simulink model "PLANTA_2019"  (R2020a)
settings: Solver=FixedStepAuto  StartTime=0.0  StopTime=10  FixedStep=0.1  RelTol=1e-3
libraries: simulink x1
settings Model: SimulationMode=accelerator  Creator=Alex  LastModifiedBy=marco
settings SFSimCC: CustomCodeUndefinedFunction=UseInterfaceOnly

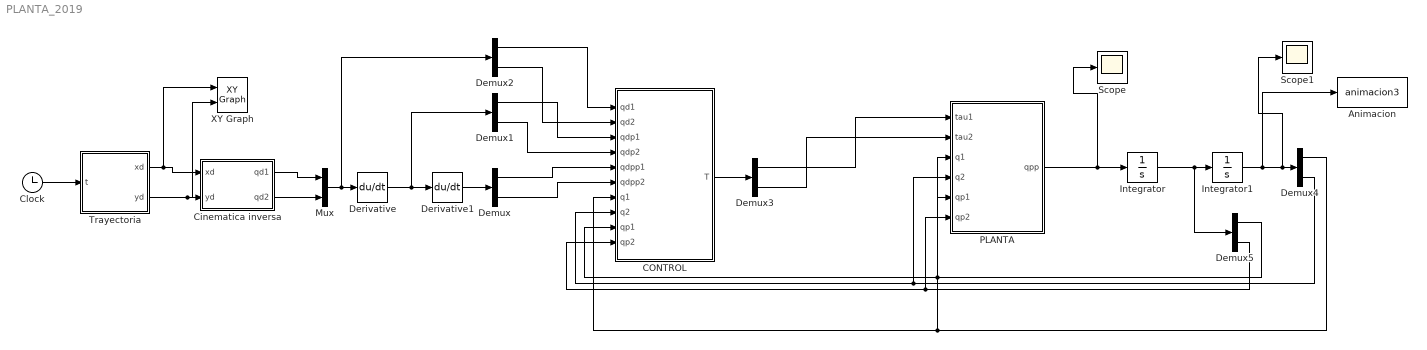
== system PLANTA_2019 ==
  Animacion : MATLABFcn  MATLABFcn=animacion3  OutputDimensions=0
  CONTROL : MATLAB Function  TreatAsAtomicUnit=on
  Cinematica inversa : MATLAB Function  TreatAsAtomicUnit=on
  Clock : Clock
  Demux{,1..5} (6 alike) : Demux  Outputs=2
  Derivative : Derivative
  Derivative1 : Derivative
  Integrator : Integrator  InitialCondition=[0 0]
  Integrator1 : Integrator  InitialCondition=[0 0]
  Mux : Mux  Inputs=2
  PLANTA : MATLAB Function  TreatAsAtomicUnit=on
  Scope : Scope
  Scope1 : Scope
  Trayectoria : MATLAB Function  TreatAsAtomicUnit=on
  XY Graph : simulink/Sinks/XY Graph  xmin=-1  xmax=1  ymin=-1  ymax=1  st=-1
  wires:
  PLANTA/1(qpp) -> Scope/1, Integrator/1
  Integrator/1 -> Demux5/1, Integrator1/1
  Clock/1 -> Trayectoria/1(t)
  Trayectoria/2(yd) -> XY Graph/2, Cinematica inversa/2(yd)
  Trayectoria/1(xd) -> Cinematica inversa/1(xd), XY Graph/1
  Cinematica inversa/1(qd1) -> Mux/1
  Mux/1 -> Demux2/1, Derivative/1
  Derivative/1 -> Demux1/1, Derivative1/1
  Derivative1/1 -> Demux/1
  Demux/1 -> CONTROL/5(qdpp1)
  Demux/2 -> CONTROL/6(qdpp2)
  Demux1/1 -> CONTROL/3(qdp1)
  Demux1/2 -> CONTROL/4(qdp2)
  Demux2/1 -> CONTROL/1(qd1)
  Demux2/2 -> CONTROL/2(qd2)
  CONTROL/1(T) -> Demux3/1
  Demux3/1 -> PLANTA/1(tau1)
  Demux3/2 -> PLANTA/2(tau2)
  Demux4/1 -> PLANTA/3(q1), CONTROL/7(q1)
  Demux4/2 -> PLANTA/4(q2), CONTROL/8(q2)
  Demux5/1 -> PLANTA/5(qp1), CONTROL/9(qp1)
  Demux5/2 -> PLANTA/6(qp2), CONTROL/10(qp2)
  Integrator1/1 -> Animacion/1, Scope1/1, Demux4/1
  Cinematica inversa/2(qd2) -> Mux/2

== matlab function PLANTA_2019/Trayectoria ==
  data: t input; xd output; yd output
function [xd,yd] = fcn(t)
% a=0.15;
% R=0.2;
% n=3;
% hx=0.3;
% hy=0.1;
% T=10;
% f=1/T;
% w=2*pi*f;
% xd=hx+(a+R*cos(n*w*t)^2)*cos(w*t);
% yd=hy+(a+R*cos(n*w*t)^2)*sin(w*t);

a=0.15;
R=0.2;
hx=0.2;
hy=0;
T=10;
f=1/T;
w=2*pi*f;
xd=hx+a*cos(w*t)/(1+sin(w*t)^2);
yd=hy+a*sin(w*t)*cos(w*t)/(1+sin(w*t)^2);

== matlab function PLANTA_2019/PLANTA ==
  data: tau1 input; qpp output; tau2 input; q1 input; q2 input; qp1 input; qp2 input
function qpp = fcn(tau1,tau2,q1,q2,qp1,qp2)
%Parámetros del primer eslabon

m1 = 0.067  %Masa de la barra 1(kg)
m2 =0.067  %Masa de la barra 2 (kg)
l1 = 0.3  % Longitud de la barra 1 (m)
lc1 = 0.14  % Longitud al centro de masa de la barra 2 (m)

l2= 0.3 %0Longitud de la baraa 2 (m)
lc2=0.15 %Longitud al centro de masa de la barra 2(m)
b1 = 0.0017  % Coeficiente de fricción viscosa de la barra 1
b2= 0.0013 %Coeficiente de fricción viscosa de la barra 2
g = 9.81  % Aceleración de la gravedad en la Tierra
I1 = 0.15  % Tensor de inercia del péndulo 1
I2= 0.14 %Tensor de inercia del péndulo 2

%Matriz de masas
M11=m1*lc1^2+m2*l2^2+m2*lc2^2+2*m2*l1*lc2*cos(q2)+I1+I2;
M12=m2*lc2^2+m2*l1*lc2*cos(q2)+I2;
M21=m2*lc2^2+m2*l1*lc2*cos(q2)+I2;
M22=m2*lc2^2+I2;
M=[M11 M12;M21 M22];

%Matriz de Coriollis
C11=-2*m2*l1*lc2*sin(q2)*qp2;
C12=-m2*l1*lc2*sin(q2)*qp2;
C21=m2*l1*lc2*sin(q2)*qp1;
C22=0
C=[C11 C12;C21 C22];

B11=b1;
B12=0;
B21=0;
B22=b2;
B=[B11 B12;B21 B22];

%Vector de gravedad
G1=(m1*lc1+m2*l1)*g*sin(q1)+m2*g*lc2*sin(q1+q2);
G2=m2*g*lc2*sin(q1+q2);

G=[G1;G2];

%Vector de posicion
q=[q1;q2];

%Vector de velocidad
qp=[qp1;qp2];

%Vector de entradas
%tau1=10;tau2=2;
T=[tau1;tau2]


%Planta

qpp = M\(T-C*qp-B*qp-G);

== matlab function PLANTA_2019/Cinematica inversa ==
  data: xd input; qd1 output; yd input; qd2 output
function [qd1,qd2] = fcn(xd,yd)
l1=0.3;
l2=0.3;
cosq2=(xd^2+yd^2-l1^2-l2^2)/(2*l1*l2);
qd2=atan2(sqrt(1-cosq2^2),cosq2);

qd1 = atan2(xd,-yd)-atan2(l2*sin(qd2),(l1+l2*cos(qd2)));

== matlab function PLANTA_2019/CONTROL ==
  data: qd1 input; T output; qd2 input; qdp1 input; qdp2 input; qdpp1 input; qdpp2 input; q1 input; q2 input; qp1 input; qp2 input
function T = fcn(qd1,qd2,qdp1,qdp2,qdpp1,qdpp2,q1,q2,qp1,qp2)
%Control por par calculado

m1 = 0.067  %Masa de la barra 1(kg)
m2 =0.067  %Masa de la barra 2 (kg)
l1 = 0.3  % Longitud de la barra 1 (m)
lc1 = 0.14  % Longitud al centro de masa de la barra 2 (m)

l2= 0.3 %0Longitud de la baraa 2 (m)
lc2=0.15 %Longitud al centro de masa de la barra 2(m)
b1 = 0.0017  % Coeficiente de fricción viscosa de la barra 1
b2= 0.0013 %Coeficiente de fricción viscosa de la barra 2
g = 9.81  % Aceleración de la gravedad en la Tierra
I1 = 0.15  % Tensor de inercia del péndulo 1
I2= 0.14 %Tensor de inercia del péndulo 2

%Matriz de masas
M11=m1*lc1^2+m2*l2^2+m2*lc2^2+2*m2*l1*lc2*cos(q2)+I1+I2;
M12=m2*lc2^2+m2*l1*lc2*cos(q2)+I2;
M21=m2*lc2^2+m2*l1*lc2*cos(q2)+I2;
M22=m2*lc2^2+I2;
M=[M11 M12;M21 M22];

%Matriz de Coriollis
C11=-2*m2*l1*lc2*sin(q2)*qp2;
C12=-m2*l1*lc2*sin(q2)*qp2;
C21=m2*l1*lc2*sin(q2)*qp1;
C22=0
C=[C11 C12;C21 C22];

B11=b1;
B12=0;
B21=0;
B22=b2;
B=[B11 B12;B21 B22];

%Vector de gravedad
G1=(m1*lc1+m2*l1)*g*sin(q1)+m2*g*lc2*sin(q1+q2);
G2=m2*g*lc2*sin(q1+q2);

G=[G1;G2];

%Vector de posicion
q=[q1;q2];

%Vector de velocidad
qp=[qp1;qp2];


kp1=15;
kp2=5;
kd1=3;
kd2=4;

%Ganancias

Kp11=kp1;
Kp12=0;
Kp21=0;
Kp22=kp2;
Kp=[Kp11 Kp12;Kp21 Kp22];

Kd11=kd1;
Kd12=0;
Kd21=0;
Kd22=kd2;
Kd=[Kd11 Kd12;Kd21 Kd22];

%Vector error de posicion
qh=[qd1-q1;qd2-q2];

%Vector de velocidad
qp=[qp1;qp2];

%Vector de aceleración
qdpp=[qdpp1;qdpp2];

%Vector de error de velocidad
qhp=[qdp1-qp1;qdp2-qp2]



T = M*(qdpp+Kd*qhp+Kp*qh)+C*qp+B*qp+G;
